simulink model "bhzzz"  (R2016b)
settings: Solver=ode15s  StartTime=0.0  StopTime=60  FixedStep=0.001  RelTol=1e-5  EnableMultiTasking=on
undefined symbols (not defined in the file): b1_damp, b2_damp, b3_damp, b4_damp, g, Hz, L1x, L1y, L1z, L2x, L2y, L2z, L3x, L3y, L3z, mass1, mass2, mass3, mass4, Rturn, theta1_0, theta1_dot_0, theta2_0, theta2_dot_0, theta3_0, theta3_dot_0, theta4_0, theta4_dot_0, X, Y, Z
libraries: sm_lib x50, nesl_utility x34, simulink_extras x2, discretizing x1, simulink x1
(part 2 of 4)

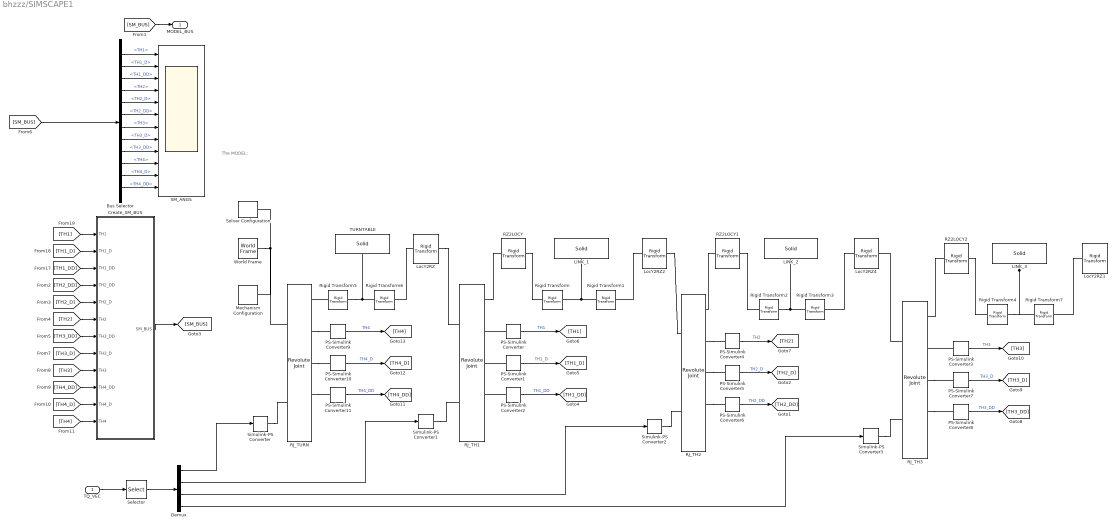
== system bhzzz/SIMSCAPE1 ==
  note: The MODEL:
  TQ_VEC : Inport
  Bus Selector : BusSelector  OutputSignals=TH1,TH1_D,TH1_DD,TH2,TH2_D,TH2_DD,TH3,TH3_D,TH3_DD,TH4,TH4_D,TH4_DD
  Create_SM_BUS : Subsystem
  Demux : Demux
  LINK_1 : sm_lib/Body Elements/Solid  InertiaType=CalculateFromGeometry  Mass=1  MassUnits=kg  CenterOfMass=[0 0 0]  CenterOfMassUnits=m  MomentsOfInertia=[1 1 1]  MomentsOfInertiaUnits=kg*m^2  ProductsOfInertia=[0 0 0]  ProductsOfInertiaUnits=kg*m^2  DensityBased=on  Density=density  DensityUnits=kg/(m^3)  DoExposeReferenceFrame=on  SerializedFrames=<Frames/>  GraphicType=FromGeometry  MarkerShape=Sphere  MarkerSize=10  GraphicVisPropType=SimpleVisualProperties  GraphicDiffuseColor=[0.2 0.2 1.0]  GraphicSpecularColor=[0.5 0.5 0.5 1.0]  GraphicAmbientColor=[0.15 0.15 0.15 1.0]  GraphicEmissiveColor=[0.0 0.0 0.0 1.0]  GraphicShininess=75  GraphicOpacity=1.0  GeometryShape=Brick  RectangleSize=[1 1]  RectangleSizeUnits=m  BrickDimensions=[L1x, L1y, L1z ]  BrickDimensionUnits=m  CylinderRadius=1  CylinderRadiusUnits=m  CylinderLength=1  CylinderLengthUnits=m  SphereRadius=1  SphereRadiusUnits=m  EllipsoidRadii=[1 1 1]  EllipsoidRadiiUnits=m  ExtrusionCrossSection=[1 1; -1 1; -1 -1; 1 -1]  ExtrusionCrossSectionUnits=m  ExtrusionLength=1  ExtrusionLengthUnits=m  PolygonNumSides=3  PolygonOuterRadius=1  PolygonOuterRadiusUnits=m  ExtGeomFileType=STEP  ExtGeomFileUnits=m  RevolutionCrossSection=[1 1; 1 -1; 2 -1; 2 1]  RevolutionCrossSectionUnits=m  RevolutionExtent=Full  RevolutionAngle=180  RevolutionAngleUnits=deg
  LINK_2 : sm_lib/Body Elements/Solid  InertiaType=CalculateFromGeometry  Mass=1  MassUnits=kg  CenterOfMass=[0 0 0]  CenterOfMassUnits=m  MomentsOfInertia=[1 1 1]  MomentsOfInertiaUnits=kg*m^2  ProductsOfInertia=[0 0 0]  ProductsOfInertiaUnits=kg*m^2  DensityBased=on  Density=density  DensityUnits=kg/(m^3)  DoExposeReferenceFrame=on  SerializedFrames=<Frames/>  GraphicType=FromGeometry  MarkerShape=Sphere  MarkerSize=10  GraphicVisPropType=SimpleVisualProperties  GraphicDiffuseColor=[0.8 0.8 1.0]  GraphicSpecularColor=[0.5 0.5 0.5 1.0]  GraphicAmbientColor=[0.15 0.15 0.15 1.0]  GraphicEmissiveColor=[0.0 0.0 0.0 1.0]  GraphicShininess=75  GraphicOpacity=1.0  GeometryShape=Brick  RectangleSize=[1 1]  RectangleSizeUnits=m  BrickDimensions=[L2x, L2y, L2z ]  BrickDimensionUnits=m  CylinderRadius=1  CylinderRadiusUnits=m  CylinderLength=1  CylinderLengthUnits=m  SphereRadius=1  SphereRadiusUnits=m  EllipsoidRadii=[1 1 1]  EllipsoidRadiiUnits=m  ExtrusionCrossSection=[1 1; -1 1; -1 -1; 1 -1]  ExtrusionCrossSectionUnits=m  ExtrusionLength=1  ExtrusionLengthUnits=m  PolygonNumSides=3  PolygonOuterRadius=1  PolygonOuterRadiusUnits=m  ExtGeomFileType=STEP  ExtGeomFileUnits=m  RevolutionCrossSection=[1 1; 1 -1; 2 -1; 2 1]  RevolutionCrossSectionUnits=m  RevolutionExtent=Full  RevolutionAngle=180  RevolutionAngleUnits=deg
  LINK_3 : sm_lib/Body Elements/Solid  InertiaType=CalculateFromGeometry  Mass=1  MassUnits=kg  CenterOfMass=[0 0 0]  CenterOfMassUnits=m  MomentsOfInertia=[1 1 1]  MomentsOfInertiaUnits=kg*m^2  ProductsOfInertia=[0 0 0]  ProductsOfInertiaUnits=kg*m^2  DensityBased=on  Density=density  DensityUnits=kg/(m^3)  DoExposeReferenceFrame=on  SerializedFrames=<Frames/>  GraphicType=FromGeometry  MarkerShape=Sphere  MarkerSize=10  GraphicVisPropType=SimpleVisualProperties  GraphicDiffuseColor=[1.0 0.8 0.4]  GraphicSpecularColor=[0.5 0.5 0.5 1.0]  GraphicAmbientColor=[0.15 0.15 0.15 1.0]  GraphicEmissiveColor=[0.0 0.0 0.0 1.0]  GraphicShininess=75  GraphicOpacity=1.0  GeometryShape=Brick  RectangleSize=[1 1]  RectangleSizeUnits=m  BrickDimensions=[L3x, L3y, L3z ]  BrickDimensionUnits=m  CylinderRadius=1  CylinderRadiusUnits=m  CylinderLength=1  CylinderLengthUnits=m  SphereRadius=1  SphereRadiusUnits=m  EllipsoidRadii=[1 1 1]  EllipsoidRadiiUnits=m  ExtrusionCrossSection=[1 1; -1 1; -1 -1; 1 -1]  ExtrusionCrossSectionUnits=m  ExtrusionLength=1  ExtrusionLengthUnits=m  PolygonNumSides=3  PolygonOuterRadius=1  PolygonOuterRadiusUnits=m  ExtGeomFileType=STEP  ExtGeomFileUnits=m  RevolutionCrossSection=[1 1; 1 -1; 2 -1; 2 1]  RevolutionCrossSectionUnits=m  RevolutionExtent=Full  RevolutionAngle=180  RevolutionAngleUnits=deg
  LocY2RZ{,1..2,4} (4 alike) : sm_lib/Frames and Transforms/Rigid Transform  TranslationMethod=None  TranslationStandardOffset=Hz/2  TranslationLengthUnit=m  TranslationStandardAxis=+Z  TranslationCartesianOffset=[0 0 0]  TranslationROffset=0  TranslationROffsetUnits=m  TranslationZOffset=0  TranslationZOffsetUnits=m  TranslationThetaOffset=0  TranslationThetaOffsetUnits=deg  RotationMethod=AlignedAxes  RotationAngleUnits=deg  RotationStandardAxis=+Z  RotationAngle=0.0  RotationArbitraryAxis=[0 0 1]  FollAlignAxisA=+X  BaseAlignAxisA=+Y  FollAlignAxisB=+Y  BaseAlignAxisB=+Z  RotationSequenceAxes=FollowerAxes  RotationSequence=XYX  RotationSequenceAngles=[0 0 0]  RotationSequenceAnglesUnits=deg  RotationMatrix=[1 0 0; 0 1 0; 0 0 1]
  Mechanism Configuration : sm_lib/Utilities/Mechanism Configuration  UniformGravity=Constant  GravityVector=[0 0 -9.80665 ]  GravityUnits=m/s^2  LinearizationDelta=1e-4
  PS-Simulink Converter{,3..4,9} (4 alike) : nesl_utility/PS-Simulink Converter  PhysicalDomain=network_engine_domain  SubClassName=ps_output  LeftPortType=input  RightPortType=output  PseudoPeriodic=off  Frequencies=[]  Unit=rad  AffineConversion=off
  PS-Simulink Converter{1,5,7,10} (4 alike) : nesl_utility/PS-Simulink Converter  PhysicalDomain=network_engine_domain  SubClassName=ps_output  LeftPortType=input  RightPortType=output  PseudoPeriodic=off  Frequencies=[]  Unit=rad/s  AffineConversion=off
  PS-Simulink Converter{2,6,8,11} (4 alike) : nesl_utility/PS-Simulink Converter  PhysicalDomain=network_engine_domain  SubClassName=ps_output  LeftPortType=input  RightPortType=output  PseudoPeriodic=off  Frequencies=[]  Unit=rad/s^2  AffineConversion=off
  RJ_TH1 : sm_lib/Joints/Revolute Joint  SenseConstraintForce=on  SenseConstraintForceX=off  SenseConstraintForceY=off  SenseConstraintForceZ=off  SenseConstraintTorque=off  SenseConstraintTorqueX=off  SenseConstraintTorqueY=off  SenseConstraintTorqueZ=off  SenseTotalForce=off  SenseTotalForceX=off  SenseTotalForceY=off  SenseTotalForceZ=off  SenseTotalTorque=off  SenseTotalTorqueX=off  SenseTotalTorqueY=off  SenseTotalTorqueZ=off  CompositeWrenchDir=BaseOnFollower  CompositeWrenchFrame=BaseFrame  EquilibriumPosition=0  EquilibriumPositionUnits=deg  SpringStiffness=0  SpringStiffnessUnits=N*m/deg  DampingCoefficient=b1_damp  DampingCoefficientUnits=N*m/(rad/s)  TorqueActuationMode=InputTorque  MotionActuationMode=ComputedMotion  SensePosition=on  SenseVelocity=on  SenseAcceleration=on  SenseTorqueForce=off  PositionTargetSpecify=on  PositionTargetPriority=Low  PositionTargetValue=theta1_0  PositionTargetValueUnits=rad  VelocityTargetSpecify=on  VelocityTargetPriority=High  VelocityTargetValue=theta1_dot_0  VelocityTargetValueUnits=rad/s
      settings: AttributesFormatString=|
      | %<DampingCoefficient>
      | %<PositionTargetValue>
      | %<VelocityTargetValue>
  RJ_TH2 : sm_lib/Joints/Revolute Joint  SenseConstraintForce=on  SenseConstraintForceX=off  SenseConstraintForceY=off  SenseConstraintForceZ=off  SenseConstraintTorque=off  SenseConstraintTorqueX=off  SenseConstraintTorqueY=off  SenseConstraintTorqueZ=off  SenseTotalForce=off  SenseTotalForceX=off  SenseTotalForceY=off  SenseTotalForceZ=off  SenseTotalTorque=off  SenseTotalTorqueX=off  SenseTotalTorqueY=off  SenseTotalTorqueZ=off  CompositeWrenchDir=BaseOnFollower  CompositeWrenchFrame=BaseFrame  EquilibriumPosition=0  EquilibriumPositionUnits=deg  SpringStiffness=0  SpringStiffnessUnits=N*m/deg  DampingCoefficient=b2_damp  DampingCoefficientUnits=N*m/(rad/s)  TorqueActuationMode=InputTorque  MotionActuationMode=ComputedMotion  SensePosition=on  SenseVelocity=on  SenseAcceleration=on  SenseTorqueForce=off  PositionTargetSpecify=on  PositionTargetPriority=Low  PositionTargetValue=theta2_0  PositionTargetValueUnits=rad  VelocityTargetSpecify=on  VelocityTargetPriority=High  VelocityTargetValue=theta2_dot_0  VelocityTargetValueUnits=rad/s
      settings: AttributesFormatString=|
      | %<DampingCoefficient>
      | %<PositionTargetValue>
      | %<VelocityTargetValue>
  RJ_TH3 : sm_lib/Joints/Revolute Joint  SenseConstraintForce=on  SenseConstraintForceX=off  SenseConstraintForceY=off  SenseConstraintForceZ=off  SenseConstraintTorque=off  SenseConstraintTorqueX=off  SenseConstraintTorqueY=off  SenseConstraintTorqueZ=off  SenseTotalForce=off  SenseTotalForceX=off  SenseTotalForceY=off  SenseTotalForceZ=off  SenseTotalTorque=off  SenseTotalTorqueX=off  SenseTotalTorqueY=off  SenseTotalTorqueZ=off  CompositeWrenchDir=BaseOnFollower  CompositeWrenchFrame=BaseFrame  EquilibriumPosition=0  EquilibriumPositionUnits=deg  SpringStiffness=0  SpringStiffnessUnits=N*m/deg  DampingCoefficient=b3_damp  DampingCoefficientUnits=N*m/(rad/s)  TorqueActuationMode=InputTorque  MotionActuationMode=ComputedMotion  SensePosition=on  SenseVelocity=on  SenseAcceleration=on  SenseTorqueForce=off  PositionTargetSpecify=on  PositionTargetPriority=Low  PositionTargetValue=theta3_0  PositionTargetValueUnits=rad  VelocityTargetSpecify=on  VelocityTargetPriority=High  VelocityTargetValue=theta3_dot_0  VelocityTargetValueUnits=rad/s
      settings: AttributesFormatString=|
      | %<DampingCoefficient>
      | %<PositionTargetValue>
      | %<VelocityTargetValue>
  RJ_TURN : sm_lib/Joints/Revolute Joint  SenseConstraintForce=on  SenseConstraintForceX=off  SenseConstraintForceY=off  SenseConstraintForceZ=off  SenseConstraintTorque=off  SenseConstraintTorqueX=off  SenseConstraintTorqueY=off  SenseConstraintTorqueZ=off  SenseTotalForce=off  SenseTotalForceX=off  SenseTotalForceY=off  SenseTotalForceZ=off  SenseTotalTorque=off  SenseTotalTorqueX=off  SenseTotalTorqueY=off  SenseTotalTorqueZ=off  CompositeWrenchDir=BaseOnFollower  CompositeWrenchFrame=BaseFrame  EquilibriumPosition=0  EquilibriumPositionUnits=deg  SpringStiffness=0  SpringStiffnessUnits=N*m/deg  DampingCoefficient=b4_damp  DampingCoefficientUnits=N*m/(rad/s)  TorqueActuationMode=InputTorque  MotionActuationMode=ComputedMotion  SensePosition=on  SenseVelocity=on  SenseAcceleration=on  SenseTorqueForce=off  PositionTargetSpecify=on  PositionTargetPriority=Low  PositionTargetValue=theta4_0  PositionTargetValueUnits=rad  VelocityTargetSpecify=on  VelocityTargetPriority=High  VelocityTargetValue=theta4_dot_0  VelocityTargetValueUnits=rad/s
      settings: AttributesFormatString=|
      | %<DampingCoefficient>
      | %<PositionTargetValue>
      | %<VelocityTargetValue>
  RZ2LOCY : sm_lib/Frames and Transforms/Rigid Transform  TranslationMethod=None  TranslationStandardOffset=Hz/2  TranslationLengthUnit=m  TranslationStandardAxis=+Z  TranslationCartesianOffset=[0 0 0]  TranslationROffset=0  TranslationROffsetUnits=m  TranslationZOffset=0  TranslationZOffsetUnits=m  TranslationThetaOffset=0  TranslationThetaOffsetUnits=deg  RotationMethod=AlignedAxes  RotationAngleUnits=deg  RotationStandardAxis=+Z  RotationAngle=0.0  RotationArbitraryAxis=[0 0 1]  FollAlignAxisA=+Y  BaseAlignAxisA=+X  FollAlignAxisB=+X  BaseAlignAxisB=+Z  RotationSequenceAxes=FollowerAxes  RotationSequence=XYX  RotationSequenceAngles=[0 0 0]  RotationSequenceAnglesUnits=deg  RotationMatrix=[1 0 0; 0 1 0; 0 0 1]
  RZ2LOCY1 : sm_lib/Frames and Transforms/Rigid Transform  TranslationMethod=None  TranslationStandardOffset=Hz/2  TranslationLengthUnit=m  TranslationStandardAxis=+Z  TranslationCartesianOffset=[0 0 0]  TranslationROffset=0  TranslationROffsetUnits=m  TranslationZOffset=0  TranslationZOffsetUnits=m  TranslationThetaOffset=0  TranslationThetaOffsetUnits=deg  RotationMethod=AlignedAxes  RotationAngleUnits=deg  RotationStandardAxis=+Z  RotationAngle=0.0  RotationArbitraryAxis=[0 0 1]  FollAlignAxisA=+Y  BaseAlignAxisA=+X  FollAlignAxisB=+X  BaseAlignAxisB=+Z  RotationSequenceAxes=FollowerAxes  RotationSequence=XYX  RotationSequenceAngles=[0 0 0]  RotationSequenceAnglesUnits=deg  RotationMatrix=[1 0 0; 0 1 0; 0 0 1]
  RZ2LOCY2 : sm_lib/Frames and Transforms/Rigid Transform  TranslationMethod=None  TranslationStandardOffset=Hz/2  TranslationLengthUnit=m  TranslationStandardAxis=+Z  TranslationCartesianOffset=[0 0 0]  TranslationROffset=0  TranslationROffsetUnits=m  TranslationZOffset=0  TranslationZOffsetUnits=m  TranslationThetaOffset=0  TranslationThetaOffsetUnits=deg  RotationMethod=AlignedAxes  RotationAngleUnits=deg  RotationStandardAxis=+Z  RotationAngle=0.0  RotationArbitraryAxis=[0 0 1]  FollAlignAxisA=+Y  BaseAlignAxisA=+X  FollAlignAxisB=+X  BaseAlignAxisB=+Z  RotationSequenceAxes=FollowerAxes  RotationSequence=XYX  RotationSequenceAngles=[0 0 0]  RotationSequenceAnglesUnits=deg  RotationMatrix=[1 0 0; 0 1 0; 0 0 1]
  Rigid Transform : sm_lib/Frames and Transforms/Rigid Transform  TranslationMethod=StandardAxis  TranslationStandardOffset=L1y/2  TranslationLengthUnit=m  TranslationStandardAxis=+Y  TranslationCartesianOffset=[0 0 0]  TranslationROffset=0  TranslationROffsetUnits=m  TranslationZOffset=0  TranslationZOffsetUnits=m  TranslationThetaOffset=0  TranslationThetaOffsetUnits=deg  RotationMethod=None  RotationAngleUnits=deg  RotationStandardAxis=+Z  RotationAngle=0.0  RotationArbitraryAxis=[0 0 1]  FollAlignAxisA=+X  BaseAlignAxisA=+Y  FollAlignAxisB=+Y  BaseAlignAxisB=+Z  RotationSequenceAxes=FollowerAxes  RotationSequence=XYX  RotationSequenceAngles=[0 0 0]  RotationSequenceAnglesUnits=deg  RotationMatrix=[1 0 0; 0 1 0; 0 0 1]
  Rigid Transform1 : sm_lib/Frames and Transforms/Rigid Transform  TranslationMethod=StandardAxis  TranslationStandardOffset=L1y/2  TranslationLengthUnit=m  TranslationStandardAxis=+Y  TranslationCartesianOffset=[0 0 0]  TranslationROffset=0  TranslationROffsetUnits=m  TranslationZOffset=0  TranslationZOffsetUnits=m  TranslationThetaOffset=0  TranslationThetaOffsetUnits=deg  RotationMethod=None  RotationAngleUnits=deg  RotationStandardAxis=+Z  RotationAngle=0.0  RotationArbitraryAxis=[0 0 1]  FollAlignAxisA=+X  BaseAlignAxisA=+Y  FollAlignAxisB=+Y  BaseAlignAxisB=+Z  RotationSequenceAxes=FollowerAxes  RotationSequence=XYX  RotationSequenceAngles=[0 0 0]  RotationSequenceAnglesUnits=deg  RotationMatrix=[1 0 0; 0 1 0; 0 0 1]
  Rigid Transform2 : sm_lib/Frames and Transforms/Rigid Transform  TranslationMethod=StandardAxis  TranslationStandardOffset=L2y/2  TranslationLengthUnit=m  TranslationStandardAxis=+Y  TranslationCartesianOffset=[0 0 0]  TranslationROffset=0  TranslationROffsetUnits=m  TranslationZOffset=0  TranslationZOffsetUnits=m  TranslationThetaOffset=0  TranslationThetaOffsetUnits=deg  RotationMethod=None  RotationAngleUnits=deg  RotationStandardAxis=+Z  RotationAngle=0.0  RotationArbitraryAxis=[0 0 1]  FollAlignAxisA=+X  BaseAlignAxisA=+Y  FollAlignAxisB=+Y  BaseAlignAxisB=+Z  RotationSequenceAxes=FollowerAxes  RotationSequence=XYX  RotationSequenceAngles=[0 0 0]  RotationSequenceAnglesUnits=deg  RotationMatrix=[1 0 0; 0 1 0; 0 0 1]
  Rigid Transform3 : sm_lib/Frames and Transforms/Rigid Transform  TranslationMethod=StandardAxis  TranslationStandardOffset=L2y/2  TranslationLengthUnit=m  TranslationStandardAxis=+Y  TranslationCartesianOffset=[0 0 0]  TranslationROffset=0  TranslationROffsetUnits=m  TranslationZOffset=0  TranslationZOffsetUnits=m  TranslationThetaOffset=0  TranslationThetaOffsetUnits=deg  RotationMethod=None  RotationAngleUnits=deg  RotationStandardAxis=+Z  RotationAngle=0.0  RotationArbitraryAxis=[0 0 1]  FollAlignAxisA=+X  BaseAlignAxisA=+Y  FollAlignAxisB=+Y  BaseAlignAxisB=+Z  RotationSequenceAxes=FollowerAxes  RotationSequence=XYX  RotationSequenceAngles=[0 0 0]  RotationSequenceAnglesUnits=deg  RotationMatrix=[1 0 0; 0 1 0; 0 0 1]
  Rigid Transform4 : sm_lib/Frames and Transforms/Rigid Transform  TranslationMethod=StandardAxis  TranslationStandardOffset=L3y/2  TranslationLengthUnit=m  TranslationStandardAxis=+Y  TranslationCartesianOffset=[0 0 0]  TranslationROffset=0  TranslationROffsetUnits=m  TranslationZOffset=0  TranslationZOffsetUnits=m  TranslationThetaOffset=0  TranslationThetaOffsetUnits=deg  RotationMethod=None  RotationAngleUnits=deg  RotationStandardAxis=+Z  RotationAngle=0.0  RotationArbitraryAxis=[0 0 1]  FollAlignAxisA=+X  BaseAlignAxisA=+Y  FollAlignAxisB=+Y  BaseAlignAxisB=+Z  RotationSequenceAxes=FollowerAxes  RotationSequence=XYX  RotationSequenceAngles=[0 0 0]  RotationSequenceAnglesUnits=deg  RotationMatrix=[1 0 0; 0 1 0; 0 0 1]
  Rigid Transform5 : sm_lib/Frames and Transforms/Rigid Transform  TranslationMethod=StandardAxis  TranslationStandardOffset=Hz/2  TranslationLengthUnit=m  TranslationStandardAxis=-Z  TranslationCartesianOffset=[0 0 0]  TranslationROffset=0  TranslationROffsetUnits=m  TranslationZOffset=0  TranslationZOffsetUnits=m  TranslationThetaOffset=0  TranslationThetaOffsetUnits=deg  RotationMethod=None  RotationAngleUnits=deg  RotationStandardAxis=+Z  RotationAngle=0.0  RotationArbitraryAxis=[0 0 1]  FollAlignAxisA=+X  BaseAlignAxisA=+Y  FollAlignAxisB=+Y  BaseAlignAxisB=+Z  RotationSequenceAxes=FollowerAxes  RotationSequence=XYX  RotationSequenceAngles=[0 0 0]  RotationSequenceAnglesUnits=deg  RotationMatrix=[1 0 0; 0 1 0; 0 0 1]
  Rigid Transform6 : sm_lib/Frames and Transforms/Rigid Transform  TranslationMethod=StandardAxis  TranslationStandardOffset=Hz/2  TranslationLengthUnit=m  TranslationStandardAxis=+Z  TranslationCartesianOffset=[0 0 0]  TranslationROffset=0  TranslationROffsetUnits=m  TranslationZOffset=0  TranslationZOffsetUnits=m  TranslationThetaOffset=0  TranslationThetaOffsetUnits=deg  RotationMethod=None  RotationAngleUnits=deg  RotationStandardAxis=+Z  RotationAngle=0.0  RotationArbitraryAxis=[0 0 1]  FollAlignAxisA=+X  BaseAlignAxisA=+Y  FollAlignAxisB=+Y  BaseAlignAxisB=+Z  RotationSequenceAxes=FollowerAxes  RotationSequence=XYX  RotationSequenceAngles=[0 0 0]  RotationSequenceAnglesUnits=deg  RotationMatrix=[1 0 0; 0 1 0; 0 0 1]
  Rigid Transform7 : sm_lib/Frames and Transforms/Rigid Transform  TranslationMethod=StandardAxis  TranslationStandardOffset=L3y/2  TranslationLengthUnit=m  TranslationStandardAxis=+Y  TranslationCartesianOffset=[0 0 0]  TranslationROffset=0  TranslationROffsetUnits=m  TranslationZOffset=0  TranslationZOffsetUnits=m  TranslationThetaOffset=0  TranslationThetaOffsetUnits=deg  RotationMethod=None  RotationAngleUnits=deg  RotationStandardAxis=+Z  RotationAngle=0.0  RotationArbitraryAxis=[0 0 1]  FollAlignAxisA=+X  BaseAlignAxisA=+Y  FollAlignAxisB=+Y  BaseAlignAxisB=+Z  RotationSequenceAxes=FollowerAxes  RotationSequence=XYX  RotationSequenceAngles=[0 0 0]  RotationSequenceAnglesUnits=deg  RotationMatrix=[1 0 0; 0 1 0; 0 0 1]
  SM_ANGS : Scope  NumInputPorts=12
  Selector : Selector  InputPortWidth=4  IndexOptions=Index vector (dialog)  Indices=[4 1 2 3]  OutputSizes=1
  Simulink-PS Converter{,1..3} (4 alike) : nesl_utility/Simulink-PS Converter  PhysicalDomain=network_engine_domain  SubClassName=ps_input  LeftPortType=input  RightPortType=output  PseudoPeriodic=off  Frequencies=[]  NoiseDistribution=none  NoiseParameters=[]  Unit=N*m  AffineConversion=off  InputFiltering=off  SimscapeFilterOrder=1  InputFilterTimeConstant=0.001  UdotUserProvided=1
  Solver Configuration : nesl_utility/Solver Configuration  PhysicalDomain=network_engine_domain  SubClassName=solver  LeftPortType=input  RightPortType=generic  Accelerate=off  Tones=[]  Harmonics=[]  SimulateNoise=off  Profile=off  UseLocalSampling=off  EnableSwitchedLinearOptims=on  FrequencyDomain=off  UseCCode=off  RelTol=0.001  AbsTol=1e-06  MinStep=1e-09  ToWorkspace=off  RevertToSquareIcSolve=off  NumHomotopyIterations=100  PhasorMode=off  PhasorModeNumHarmonics=1  OverrideAbsTol=off  DoDC=off  ResidualTolerance=1e-09  UseLocalSolver=off  LocalSolverChoice=NE_TRAPEZOIDAL_ADVANCER  LocalSolverSampleTime=0.01  DoFixedCost=off  MaxNonlinIter=3  MaxModeIter=2  LinearAlgebra=Sparse  DelaysMemoryBudget=1024  AutomaticFiltering=off  FilteringTimeConstant=0.001
  TURNTABLE : sm_lib/Body Elements/Solid  InertiaType=CalculateFromGeometry  Mass=1  MassUnits=kg  CenterOfMass=[0 0 0]  CenterOfMassUnits=m  MomentsOfInertia=[1 1 1]  MomentsOfInertiaUnits=kg*m^2  ProductsOfInertia=[0 0 0]  ProductsOfInertiaUnits=kg*m^2  DensityBased=on  Density=1000  DensityUnits=kg/(m^3)  DoExposeReferenceFrame=on  SerializedFrames=<Frames/>  GraphicType=FromGeometry  MarkerShape=Sphere  MarkerSize=10  GraphicVisPropType=SimpleVisualProperties  GraphicDiffuseColor=[1.0 1.0 0.2]  GraphicSpecularColor=[0.5 0.5 0.5 1.0]  GraphicAmbientColor=[0.15 0.15 0.15 1.0]  GraphicEmissiveColor=[0.0 0.0 0.0 1.0]  GraphicShininess=75  GraphicOpacity=1.0  GeometryShape=Cylinder  RectangleSize=[1 1]  RectangleSizeUnits=m  BrickDimensions=[1 1 1]  BrickDimensionUnits=m  CylinderRadius=Rturn  CylinderRadiusUnits=m  CylinderLength=Hz  CylinderLengthUnits=m  SphereRadius=1  SphereRadiusUnits=m  EllipsoidRadii=[1 1 1]  EllipsoidRadiiUnits=m  ExtrusionCrossSection=[1 1; -1 1; -1 -1; 1 -1]  ExtrusionCrossSectionUnits=m  ExtrusionLength=1  ExtrusionLengthUnits=m  PolygonNumSides=3  PolygonOuterRadius=1  PolygonOuterRadiusUnits=m  ExtGeomFileType=STEP  ExtGeomFileUnits=m  RevolutionCrossSection=[1 1; 1 -1; 2 -1; 2 1]  RevolutionCrossSectionUnits=m  RevolutionExtent=Full  RevolutionAngle=180  RevolutionAngleUnits=deg
  World Frame : sm_lib/Frames and Transforms/World Frame
  MODEL_BUS : Outport
  wires:
  [SM_BUS] -> MODEL_BUS/1
  [TH2_D] -> Create_SM_BUS/5(TH2_D)
  [TH1_D] -> Create_SM_BUS/2(TH1_D)
  [TH2_DD] -> Create_SM_BUS/4(TH2_DD)
  [TH2] -> Create_SM_BUS/6(TH2)
  [TH1_DD] -> Create_SM_BUS/3(TH1_DD)
  [TH1] -> Create_SM_BUS/1(TH1)
  Create_SM_BUS/1(SM_BUS) -> [SM_BUS]
  Bus Selector/2 -> SM_ANGS/2  "<TH1_D>"
  Bus Selector/3 -> SM_ANGS/3  "<TH1_DD>"
  Bus Selector/1 -> SM_ANGS/1  "<TH1>"
  Bus Selector/4 -> SM_ANGS/4  "<TH2>"
  Bus Selector/5 -> SM_ANGS/5  "<TH2_D>"
  Bus Selector/6 -> SM_ANGS/6  "<TH2_DD>"
  Bus Selector/7 -> SM_ANGS/7  "<TH3>"
  Bus Selector/8 -> SM_ANGS/8  "<TH3_D>"
  Bus Selector/9 -> SM_ANGS/9  "<TH3_DD>"
  [TH3_DD] -> Create_SM_BUS/7(TH3_DD)
  [TH3_D] -> Create_SM_BUS/8(TH3_D)
  [TH3] -> Create_SM_BUS/9(TH3)
  PS-Simulink Converter/1 -> [TH1]  "TH1"
  PS-Simulink Converter2/1 -> [TH1_DD]  "TH1_DD"
  PS-Simulink Converter1/1 -> [TH1_D]  "TH1_D"
  PS-Simulink Converter4/1 -> [TH2]  "TH2"
  PS-Simulink Converter6/1 -> [TH2_DD]  "TH2_DD"
  PS-Simulink Converter5/1 -> [TH2_D]  "TH2_D"
  PS-Simulink Converter3/1 -> [TH3]  "TH3"
  PS-Simulink Converter8/1 -> [TH3_DD]  "TH3_DD"
  PS-Simulink Converter7/1 -> [TH3_D]  "TH3_D"
  PS-Simulink Converter9/1 -> [TH4]  "TH4"
  PS-Simulink Converter11/1 -> [TH4_DD]  "TH4_DD"
  PS-Simulink Converter10/1 -> [TH4_D]  "TH4_D"
  [TH4_DD] -> Create_SM_BUS/10(TH4_DD)
  [TH4_D] -> Create_SM_BUS/11(TH4_D)
  [TH4] -> Create_SM_BUS/12(TH4)
  Bus Selector/12 -> SM_ANGS/12  "<TH4_DD>"
  Bus Selector/11 -> SM_ANGS/11  "<TH4_D>"
  Bus Selector/10 -> SM_ANGS/10  "<TH4>"
  [SM_BUS] -> Bus Selector/1
  TQ_VEC/1 -> Selector/1
  Selector/1 -> Demux/1
  Demux/1 -> Simulink-PS Converter/1
  Demux/2 -> Simulink-PS Converter1/1
  Demux/3 -> Simulink-PS Converter2/1
  Demux/4 -> Simulink-PS Converter3/1
  connections:
  World Frame/RConn1 -- RJ_TURN/LConn1 -- Mechanism Configuration/RConn1 -- Solver Configuration/RConn1
  PS-Simulink Converter1/LConn1 -- RJ_TH1/RConn3
  PS-Simulink Converter2/LConn1 -- RJ_TH1/RConn4
  PS-Simulink Converter/LConn1 -- RJ_TH1/RConn2
  Rigid Transform5/LConn1 -- RJ_TURN/RConn1
  Rigid Transform5/RConn1 -- Rigid Transform6/LConn1 -- TURNTABLE/RConn1
  LocY2RZ/LConn1 -- Rigid Transform6/RConn1
  LocY2RZ/RConn1 -- RJ_TH1/LConn1
  Rigid Transform1/LConn1 -- LINK_1/RConn1 -- Rigid Transform/RConn1
  LocY2RZ2/LConn1 -- Rigid Transform1/RConn1
  LocY2RZ2/RConn1 -- RJ_TH2/LConn1
  RZ2LOCY1/LConn1 -- RJ_TH2/RConn1
  Rigid Transform2/RConn1 -- Rigid Transform3/LConn1 -- LINK_2/RConn1
  LocY2RZ4/LConn1 -- Rigid Transform3/RConn1
  RJ_TH1/RConn1 -- RZ2LOCY/LConn1
  RZ2LOCY/RConn1 -- Rigid Transform/LConn1
  RZ2LOCY1/RConn1 -- Rigid Transform2/LConn1
  RJ_TH3/LConn1 -- LocY2RZ4/RConn1
  LINK_3/RConn1 -- Rigid Transform7/LConn1 -- Rigid Transform4/RConn1
  LocY2RZ1/LConn1 -- Rigid Transform7/RConn1
  RZ2LOCY2/RConn1 -- Rigid Transform4/LConn1
  RZ2LOCY2/LConn1 -- RJ_TH3/RConn1
  RJ_TH2/RConn3 -- PS-Simulink Converter5/LConn1
  RJ_TH2/RConn2 -- PS-Simulink Converter4/LConn1
  RJ_TH2/RConn4 -- PS-Simulink Converter6/LConn1
  PS-Simulink Converter3/LConn1 -- RJ_TH3/RConn2
  RJ_TH3/RConn3 -- PS-Simulink Converter7/LConn1
  RJ_TH3/RConn4 -- PS-Simulink Converter8/LConn1
  RJ_TURN/RConn4 -- PS-Simulink Converter11/LConn1
  RJ_TURN/RConn3 -- PS-Simulink Converter10/LConn1
  RJ_TURN/RConn2 -- PS-Simulink Converter9/LConn1
  Simulink-PS Converter/RConn1 -- RJ_TURN/LConn2
  Simulink-PS Converter2/RConn1 -- RJ_TH2/LConn2
  Simulink-PS Converter3/RConn1 -- RJ_TH3/LConn2
  Simulink-PS Converter1/RConn1 -- RJ_TH1/LConn2

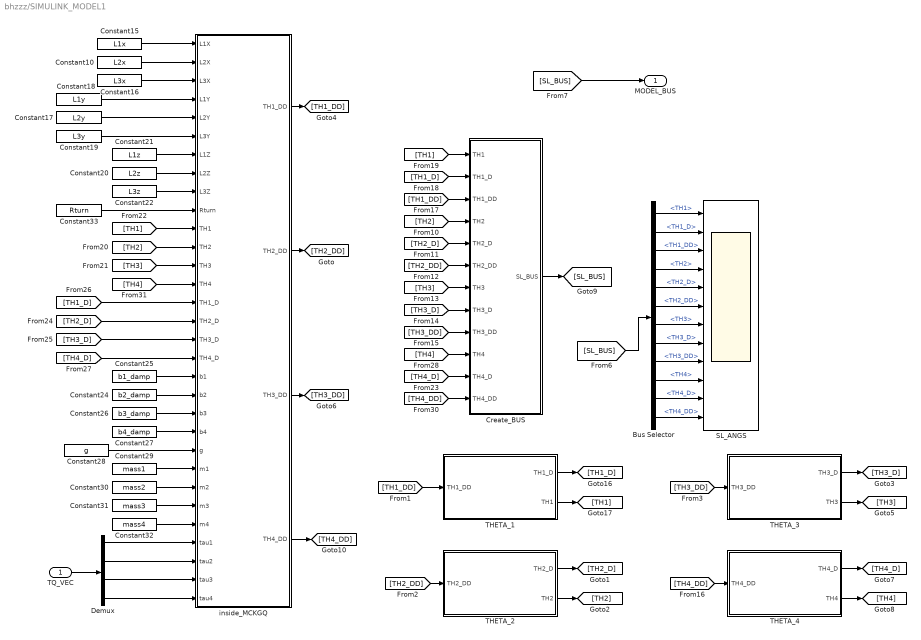
== system bhzzz/SIMULINK_MODEL1 ==
  TQ_VEC : Inport
  Bus Selector : BusSelector  OutputSignals=TH1,TH1_D,TH1_DD,TH2,TH2_D,TH2_DD,TH3,TH3_D,TH3_DD,TH4,TH4_D,TH4_DD
  Constant10 : Constant  Value=L2x
  Constant15 : Constant  Value=L1x
  Constant16 : Constant  Value=L3x
  Constant17 : Constant  Value=L2y
  Constant18 : Constant  Value=L1y
  Constant19 : Constant  Value=L3y
  Constant20 : Constant  Value=L2z
  Constant21 : Constant  Value=L1z
  Constant22 : Constant  Value=L3z
  Constant24 : Constant  Value=b2_damp
  Constant25 : Constant  Value=b1_damp
  Constant26 : Constant  Value=b3_damp
  Constant27 : Constant  Value=b4_damp
  Constant28 : Constant  Value=g
  Constant29 : Constant  Value=mass1
  Constant30 : Constant  Value=mass2
  Constant31 : Constant  Value=mass3
  Constant32 : Constant  Value=mass4
  Constant33 : Constant  Value=Rturn
  Create_BUS : Subsystem
  Demux : Demux
  SL_ANGS : Scope  NumInputPorts=12
  THETA_1 : Subsystem
  THETA_2 : Subsystem
  THETA_3 : Subsystem
  THETA_4 : Subsystem
  inside_MCKGQ : Subsystem
  MODEL_BUS : Outport
  wires:
  [SL_BUS] -> Bus Selector/1
  Create_BUS/1(SL_BUS) -> [SL_BUS]
  Bus Selector/2 -> SL_ANGS/2  "<TH1_D>"
  Bus Selector/3 -> SL_ANGS/3  "<TH1_DD>"
  Bus Selector/1 -> SL_ANGS/1  "<TH1>"
  Bus Selector/4 -> SL_ANGS/4  "<TH2>"
  Bus Selector/5 -> SL_ANGS/5  "<TH2_D>"
  Bus Selector/6 -> SL_ANGS/6  "<TH2_DD>"
  Bus Selector/7 -> SL_ANGS/7  "<TH3>"
  Bus Selector/8 -> SL_ANGS/8  "<TH3_D>"
  Bus Selector/9 -> SL_ANGS/9  "<TH3_DD>"
  [TH2_DD] -> THETA_2/1(TH2_DD)
  THETA_2/2(TH2) -> [TH2]
  THETA_2/1(TH2_D) -> [TH2_D]
  [TH1_DD] -> THETA_1/1(TH1_DD)
  THETA_1/1(TH1_D) -> [TH1_D]
  THETA_1/2(TH1) -> [TH1]
  inside_MCKGQ/2(TH2_DD) -> [TH2_DD]
  [TH3_DD] -> THETA_3/1(TH3_DD)
  THETA_3/2(TH3) -> [TH3]
  THETA_3/1(TH3_D) -> [TH3_D]
  inside_MCKGQ/1(TH1_DD) -> [TH1_DD]
  inside_MCKGQ/3(TH3_DD) -> [TH3_DD]
  [TH3_DD] -> Create_BUS/9(TH3_DD)
  [TH1] -> Create_BUS/1(TH1)
  [TH1_D] -> Create_BUS/2(TH1_D)
  [TH1_DD] -> Create_BUS/3(TH1_DD)
  [TH2] -> Create_BUS/4(TH2)
  [TH2_D] -> Create_BUS/5(TH2_D)
  [TH2_DD] -> Create_BUS/6(TH2_DD)
  [TH3] -> Create_BUS/7(TH3)
  [TH3_D] -> Create_BUS/8(TH3_D)
  [TH4_DD] -> THETA_4/1(TH4_DD)
  THETA_4/2(TH4) -> [TH4]
  THETA_4/1(TH4_D) -> [TH4_D]
  [TH2] -> inside_MCKGQ/12(TH2)
  [TH3] -> inside_MCKGQ/13(TH3)
  [TH1] -> inside_MCKGQ/11(TH1)
  Constant10/1 -> inside_MCKGQ/2(L2X)
  Constant16/1 -> inside_MCKGQ/3(L3X)
  Constant15/1 -> inside_MCKGQ/1(L1X)
  Constant19/1 -> inside_MCKGQ/6(L3Y)
  Constant17/1 -> inside_MCKGQ/5(L2Y)
  Constant18/1 -> inside_MCKGQ/4(L1Y)
  Constant22/1 -> inside_MCKGQ/9(L3Z)
  Constant20/1 -> inside_MCKGQ/8(L2Z)
  Constant21/1 -> inside_MCKGQ/7(L1Z)
  [TH1_D] -> inside_MCKGQ/15(TH1_D)
  [TH2_D] -> inside_MCKGQ/16(TH2_D)
  [TH3_D] -> inside_MCKGQ/17(TH3_D)
  [TH4_D] -> inside_MCKGQ/18(TH4_D)
  Constant25/1 -> inside_MCKGQ/19(b1)
  Constant24/1 -> inside_MCKGQ/20(b2)
  Constant26/1 -> inside_MCKGQ/21(b3)
  Constant27/1 -> inside_MCKGQ/22(b4)
  Constant28/1 -> inside_MCKGQ/23(g)
  Constant29/1 -> inside_MCKGQ/24(m1)
  Constant30/1 -> inside_MCKGQ/25(m2)
  Constant31/1 -> inside_MCKGQ/26(m3)
  Constant32/1 -> inside_MCKGQ/27(m4)
  Constant33/1 -> inside_MCKGQ/10(Rturn)
  [TH4_D] -> Create_BUS/11(TH4_D)
  [TH4_DD] -> Create_BUS/12(TH4_DD)
  [TH4] -> Create_BUS/10(TH4)
  [TH4] -> inside_MCKGQ/14(TH4)
  inside_MCKGQ/4(TH4_DD) -> [TH4_DD]
  Bus Selector/10 -> SL_ANGS/10  "<TH4>"
  Bus Selector/11 -> SL_ANGS/11  "<TH4_D>"
  Bus Selector/12 -> SL_ANGS/12  "<TH4_DD>"
  [SL_BUS] -> MODEL_BUS/1
  Demux/1 -> inside_MCKGQ/28(tau1)
  Demux/2 -> inside_MCKGQ/29(tau2)
  Demux/3 -> inside_MCKGQ/30(tau3)
  Demux/4 -> inside_MCKGQ/31(tau4)
  TQ_VEC/1 -> Demux/1

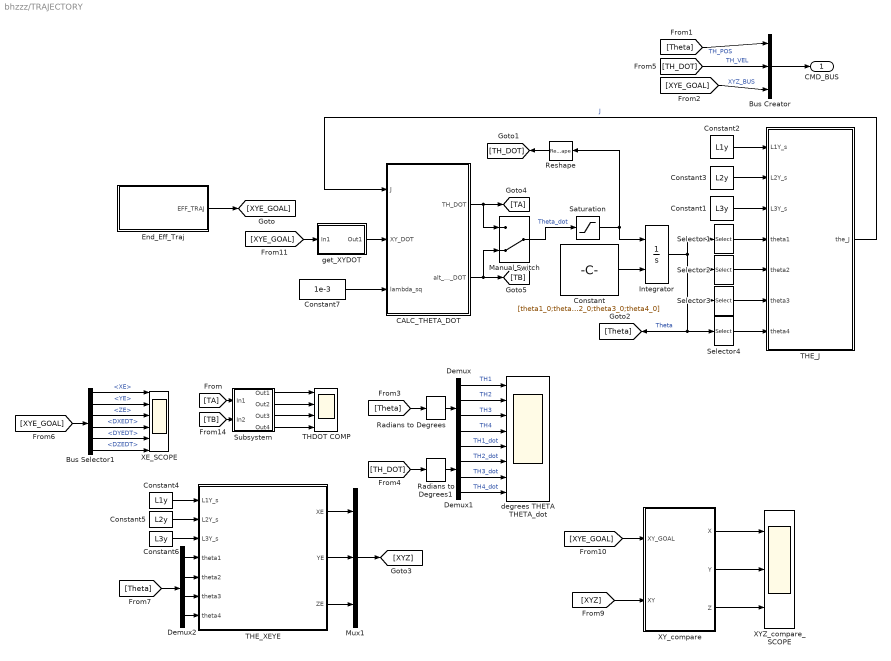
== system bhzzz/TRAJECTORY ==
  Bus Creator : BusCreator  Inputs=3
  Bus Selector1 : BusSelector  OutputSignals=XE,YE,ZE,DXEDT,DYEDT,DZEDT
  CALC_THETA_DOT : MATLAB Function  TreatAsAtomicUnit=on
  Constant : Constant  Value=[theta1_0;theta2_0;theta3_0;theta4_0]  VectorParams1D=off
  Constant1 : Constant  Value=L3y
  Constant2 : Constant  Value=L1y
  Constant3 : Constant  Value=L2y
  Constant4 : Constant  Value=L1y
  Constant5 : Constant  Value=L2y
  Constant6 : Constant  Value=L3y
  Constant7 : Constant  Value=1e-3
  Demux : Demux
  Demux1 : Demux
  Demux2 : Demux
  End_Eff_Traj : Subsystem
  Integrator : Integrator  InitialConditionSource=external
  Manual Switch : ManualSwitch  CurrentSetting=0
  Mux1 : Mux  Inputs=3
  Radians to Degrees : simulink_extras/Transformations/Radians to Degrees
  Radians to Degrees1 : simulink_extras/Transformations/Radians to Degrees
  Reshape : Reshape  OutputDimensionality=Column vector (2-D)
  Saturation : Saturate  UpperLimit=6  LowerLimit=-6
  Selector1 : Selector  InputPortWidth=4  IndexOptions=Index vector (dialog)  Indices=1  OutputSizes=1
  Selector2 : Selector  InputPortWidth=4  IndexOptions=Index vector (dialog)  Indices=2  OutputSizes=1
  Selector3 : Selector  InputPortWidth=4  IndexOptions=Index vector (dialog)  Indices=3  OutputSizes=1
  Selector4 : Selector  InputPortWidth=4  IndexOptions=Index vector (dialog)  Indices=4  OutputSizes=1
  Subsystem : Subsystem
  THDOT COMP : Scope  NumInputPorts=4
  THE_J : MATLAB Function  TreatAsAtomicUnit=on
  THE_XEYE : MATLAB Function  TreatAsAtomicUnit=on
  XE_SCOPE : Scope  NumInputPorts=6
  XYZ_compare_SCOPE : Scope  NumInputPorts=3
  XY_compare : Subsystem
  degrees THETA THETA_dot : Scope  NumInputPorts=8
  get_XYDOT : Subsystem
  CMD_BUS : Outport
  wires:
  Bus Selector1/1 -> XE_SCOPE/1  "<XE>"
  Bus Selector1/2 -> XE_SCOPE/2  "<YE>"
  Bus Selector1/3 -> XE_SCOPE/3  "<ZE>"
  Bus Selector1/4 -> XE_SCOPE/4  "<DXEDT>"
  Bus Selector1/5 -> XE_SCOPE/5  "<DYEDT>"
  Bus Selector1/6 -> XE_SCOPE/6  "<DZEDT>"
  [XYE_GOAL] -> Bus Selector1/1
  Constant/1 -> Integrator/2
  THE_J/1(the_J) -> CALC_THETA_DOT/1(J)  "J"
  get_XYDOT/1(Out1) -> CALC_THETA_DOT/2(XY_DOT)
  Manual Switch/1 -> Saturation/1  "Theta_dot"
  Integrator/1 -> Selector4/1, [Theta], Selector3/1, Selector2/1, Selector1/1  "Theta"
  [XYE_GOAL] -> get_XYDOT/1(In1)
  Saturation/1 -> Integrator/1, Reshape/1
  Selector4/1 -> THE_J/7(theta4)
  Selector3/1 -> THE_J/6(theta3)
  Selector2/1 -> THE_J/5(theta2)
  Selector1/1 -> THE_J/4(theta1)
  Constant2/1 -> THE_J/1(L1Y_s)
  Constant3/1 -> THE_J/2(L2Y_s)
  Constant1/1 -> THE_J/3(L3Y_s)
  CALC_THETA_DOT/1(TH_DOT) -> [TA], Manual Switch/1
  CALC_THETA_DOT/2(alt_TH_DOT) -> [TB], Manual Switch/2
  Constant7/1 -> CALC_THETA_DOT/3(lambda_sq)
  [TB] -> Subsystem/2(In2)
  [TA] -> Subsystem/1(In1)
  Subsystem/1(Out1) -> THDOT COMP/1
  Subsystem/2(Out2) -> THDOT COMP/2
  Subsystem/3(Out3) -> THDOT COMP/3
  Subsystem/4(Out4) -> THDOT COMP/4
  End_Eff_Traj/1(EFF_TRAJ) -> [XYE_GOAL]
  [TH_DOT] -> Bus Creator/2  "TH_VEL"
  [Theta] -> Bus Creator/1  "TH_POS"
  Bus Creator/1 -> CMD_BUS/1
  Reshape/1 -> [TH_DOT]
  [XYE_GOAL] -> Bus Creator/3  "XYZ_BUS"
  Demux/4 -> degrees THETA THETA_dot/4  "TH4"
  Demux/3 -> degrees THETA THETA_dot/3  "TH3"
  Demux/2 -> degrees THETA THETA_dot/2  "TH2"
  Demux/1 -> degrees THETA THETA_dot/1  "TH1"
  Demux1/1 -> degrees THETA THETA_dot/5  "TH1_dot"
  Demux1/2 -> degrees THETA THETA_dot/6  "TH2_dot"
  Demux1/3 -> degrees THETA THETA_dot/7  "TH3_dot"
  Demux1/4 -> degrees THETA THETA_dot/8  "TH4_dot"
  [Theta] -> Radians to Degrees/1
  Radians to Degrees/1 -> Demux/1
  [TH_DOT] -> Radians to Degrees1/1
  Radians to Degrees1/1 -> Demux1/1
  Constant4/1 -> THE_XEYE/1(L1Y_s)
  Constant6/1 -> THE_XEYE/3(L3Y_s)
  Constant5/1 -> THE_XEYE/2(L2Y_s)
  Demux2/1 -> THE_XEYE/4(theta1)
  Demux2/2 -> THE_XEYE/5(theta2)
  Demux2/3 -> THE_XEYE/6(theta3)
  Demux2/4 -> THE_XEYE/7(theta4)
  [Theta] -> Demux2/1
  THE_XEYE/1(XE) -> Mux1/1
  THE_XEYE/3(ZE) -> Mux1/3
  THE_XEYE/2(YE) -> Mux1/2
  Mux1/1 -> [XYZ]
  [XYZ] -> XY_compare/2(XY)
  XY_compare/2(Y) -> XYZ_compare_SCOPE/2
  XY_compare/1(X) -> XYZ_compare_SCOPE/1
  [XYE_GOAL] -> XY_compare/1(XY_GOAL)
  XY_compare/3(Z) -> XYZ_compare_SCOPE/3

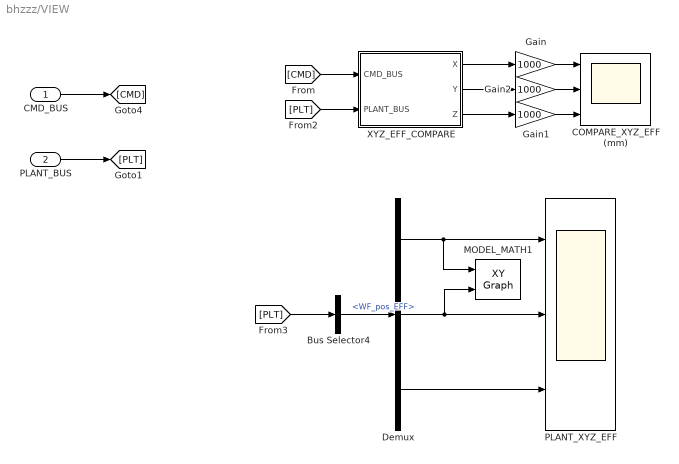
== system bhzzz/VIEW ==
  CMD_BUS : Inport
  PLANT_BUS : Inport  Port=2
  Bus Selector4 : BusSelector  OutputSignals=CALC_POS_BUS.WF_pos_EFF
  COMPARE_XYZ_EFF (mm) : Scope  NumInputPorts=3
  Demux : Demux  Outputs=3
  Gain : Gain  Gain=1000
  Gain1 : Gain  Gain=1000
  Gain2 : Gain  Gain=1000
  MODEL_MATH1 : simulink/Sinks/XY Graph  xmin=0  xmax=1.6  ymin=0  ymax=1.6  st=-1
  PLANT_XYZ_EFF : Scope  NumInputPorts=3
  XYZ_EFF_COMPARE : Subsystem
  wires:
  CMD_BUS/1 -> [CMD]
  PLANT_BUS/1 -> [PLT]
  [CMD] -> XYZ_EFF_COMPARE/1(CMD_BUS)
  [PLT] -> XYZ_EFF_COMPARE/2(PLANT_BUS)
  XYZ_EFF_COMPARE/1(X) -> Gain/1
  XYZ_EFF_COMPARE/2(Y) -> Gain2/1
  XYZ_EFF_COMPARE/3(Z) -> Gain1/1
  Bus Selector4/1 -> Demux/1  "<WF_pos_EFF>"
  Demux/1 -> MODEL_MATH1/1, PLANT_XYZ_EFF/1
  Demux/2 -> MODEL_MATH1/2, PLANT_XYZ_EFF/2
  [PLT] -> Bus Selector4/1
  Demux/3 -> PLANT_XYZ_EFF/3
  Gain/1 -> COMPARE_XYZ_EFF (mm)/1
  Gain1/1 -> COMPARE_XYZ_EFF (mm)/3
  Gain2/1 -> COMPARE_XYZ_EFF (mm)/2

== system bhzzz/Create_PLANT_BUS1/CALC_BUS ==
  MODEL_BUS : Inport
  Bus Creator : BusCreator  Inputs=14
  Bus Selector : BusSelector  OutputSignals=TH1,TH2,TH3,TH4
  Bus Selector1 : BusSelector  OutputSignals=TH1,TH2,TH3
  Constant1 : Constant  Value=L2y
  Constant17 : Constant  Value=L2y
  Constant18 : Constant  Value=L1y
  Constant19 : Constant  Value=L3y
  Constant2 : Constant  Value=L1y
  Constant3 : Constant  Value=L3y
  THE_A_EFF_and_O_and_G : MATLAB Function  TreatAsAtomicUnit=on
  THE_W_EFF_and_O_and_G : MATLAB Function  TreatAsAtomicUnit=on
  CALC_POS : Outport
  wires:
  Bus Selector/1 -> THE_W_EFF_and_O_and_G/4(theta1)  "<TH1>"
  Bus Selector/2 -> THE_W_EFF_and_O_and_G/5(theta2)  "<TH2>"
  Bus Selector/3 -> THE_W_EFF_and_O_and_G/6(theta3)  "<TH3>"
  Bus Selector/4 -> THE_W_EFF_and_O_and_G/7(theta4)  "<TH4>"
  Bus Creator/1 -> CALC_POS/1
  Constant18/1 -> THE_W_EFF_and_O_and_G/1(L1Y_s)
  Constant17/1 -> THE_W_EFF_and_O_and_G/2(L2Y_s)
  Constant19/1 -> THE_W_EFF_and_O_and_G/3(L3Y_s)
  THE_W_EFF_and_O_and_G/4(WF_pos_O3) -> Bus Creator/4  "WF_pos_O3"
  THE_W_EFF_and_O_and_G/6(WF_pos_G2) -> Bus Creator/6  "WF_pos_G2"
  THE_W_EFF_and_O_and_G/3(WF_pos_O2) -> Bus Creator/3  "WF_pos_O2"
  THE_W_EFF_and_O_and_G/7(WF_pos_G3) -> Bus Creator/7  "WF_pos_G3"
  THE_W_EFF_and_O_and_G/1(WF_pos_eff) -> Bus Creator/1  "WF_pos_EFF"
  THE_W_EFF_and_O_and_G/5(WF_pos_G1) -> Bus Creator/5  "WF_pos_G1"
  THE_W_EFF_and_O_and_G/2(WF_pos_O1) -> Bus Creator/2  "WF_pos_O1"
  MODEL_BUS/1 -> Bus Selector1/1, Bus Selector/1
  Bus Selector1/1 -> THE_A_EFF_and_O_and_G/4(theta1)  "<TH1>"
  Bus Selector1/2 -> THE_A_EFF_and_O_and_G/5(theta2)  "<TH2>"
  Bus Selector1/3 -> THE_A_EFF_and_O_and_G/6(theta3)  "<TH3>"
  Constant2/1 -> THE_A_EFF_and_O_and_G/1(L1Y_s)
  Constant1/1 -> THE_A_EFF_and_O_and_G/2(L2Y_s)
  Constant3/1 -> THE_A_EFF_and_O_and_G/3(L3Y_s)
  THE_A_EFF_and_O_and_G/7(AF_pos_G3) -> Bus Creator/14  "AF_pos_G3"
  THE_A_EFF_and_O_and_G/6(AF_pos_G2) -> Bus Creator/13  "AF_pos_G2"
  THE_A_EFF_and_O_and_G/5(AF_pos_G1) -> Bus Creator/12  "AF_pos_G1"
  THE_A_EFF_and_O_and_G/4(AF_pos_O3) -> Bus Creator/11  "AF_pos_O3"
  THE_A_EFF_and_O_and_G/3(AF_pos_O2) -> Bus Creator/10  "AF_pos_O2"
  THE_A_EFF_and_O_and_G/2(AF_pos_O1) -> Bus Creator/9  "AF_pos_O1"
  THE_A_EFF_and_O_and_G/1(AF_pos_eff) -> Bus Creator/8  "AF_pos_EFF"

== system bhzzz/Create_PLANT_BUS1/MEAS ==
  MODEL_BUS : Inport
  Bus Creator : BusCreator  Inputs=3
  Bus Selector : BusSelector  OutputSignals=TH1,TH2,TH3,TH4
  Bus Selector1 : BusSelector  OutputSignals=TH1_D,TH2_D,TH3_D,TH4_D
  Bus Selector2 : BusSelector  OutputSignals=TH1_DD,TH2_DD,TH3_DD,TH4_DD
  Mux : Mux
  Mux1 : Mux
  Mux2 : Mux
  Reshape : Reshape  OutputDimensionality=Column vector (2-D)
  Reshape1 : Reshape  OutputDimensionality=Column vector (2-D)
  Reshape2 : Reshape  OutputDimensionality=Column vector (2-D)
  MEAS : Outport
  wires:
  MODEL_BUS/1 -> Bus Selector/1, Bus Selector2/1, Bus Selector1/1
  Bus Selector/1 -> Mux/1  "<TH1>"
  Bus Selector/2 -> Mux/2  "<TH2>"
  Bus Selector/3 -> Mux/3  "<TH3>"
  Bus Selector/4 -> Mux/4  "<TH4>"
  Bus Selector1/1 -> Mux1/1  "<TH1_D>"
  Bus Selector1/2 -> Mux1/2  "<TH2_D>"
  Bus Selector1/3 -> Mux1/3  "<TH3_D>"
  Bus Selector1/4 -> Mux1/4  "<TH4_D>"
  Bus Selector2/1 -> Mux2/1  "<TH1_DD>"
  Bus Selector2/2 -> Mux2/2  "<TH2_DD>"
  Bus Selector2/3 -> Mux2/3  "<TH3_DD>"
  Bus Selector2/4 -> Mux2/4  "<TH4_DD>"
  Mux/1 -> Reshape/1  "TH_POS"
  Mux1/1 -> Reshape1/1  "TH_VEL"
  Mux2/1 -> Reshape2/1  "TH_ACC"
  Reshape/1 -> Bus Creator/1  "TH_POS"
  Reshape1/1 -> Bus Creator/2  "TH_VEL"
  Reshape2/1 -> Bus Creator/3  "TH_ACC"
  Bus Creator/1 -> MEAS/1

== system bhzzz/Create_PLANT_BUS1/Subsystem ==
  MODEL : Inport
  MEAS : Inport  Port=2
  CALC_POS : Inport  Port=3
  CALC_GRAV_TQ : Inport  Port=4
  Bus Creator : BusCreator  Inputs=4
  PLANT_B : Outport
  wires:
  MODEL/1 -> Bus Creator/1  "MODEL_BUS"
  MEAS/1 -> Bus Creator/2  "MEAS_BUS"
  CALC_POS/1 -> Bus Creator/3  "CALC_POS_BUS"
  Bus Creator/1 -> PLANT_B/1
  CALC_GRAV_TQ/1 -> Bus Creator/4  "CALC_GRAV_TQ_BUS"

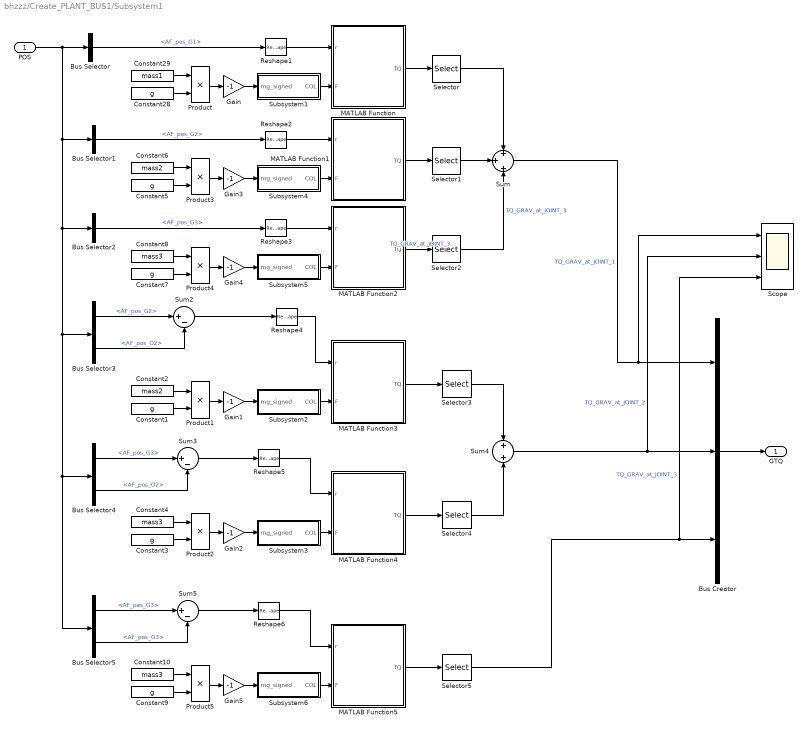
== system bhzzz/Create_PLANT_BUS1/Subsystem1 ==
  POS : Inport
  Bus Creator : BusCreator  Inputs=3
  Bus Selector : BusSelector  OutputSignals=AF_pos_G1
  Bus Selector1 : BusSelector  OutputSignals=AF_pos_G2
  Bus Selector2 : BusSelector  OutputSignals=AF_pos_G3
  Bus Selector3 : BusSelector  OutputSignals=AF_pos_G2,AF_pos_O2
  Bus Selector4 : BusSelector  OutputSignals=AF_pos_G3,AF_pos_O2
  Bus Selector5 : BusSelector  OutputSignals=AF_pos_G3,AF_pos_O3
  Constant{1,3,5,7,9,28} (6 alike) : Constant  Value=g
  Constant10 : Constant  Value=mass3
  Constant2 : Constant  Value=mass2
  Constant29 : Constant  Value=mass1
  Constant4 : Constant  Value=mass3
  Constant6 : Constant  Value=mass2
  Constant8 : Constant  Value=mass3
  Gain{,1..5} (6 alike) : Gain  Gain=-1
  MATLAB Function : MATLAB Function  TreatAsAtomicUnit=on
  MATLAB Function1 : MATLAB Function  TreatAsAtomicUnit=on
  MATLAB Function2 : MATLAB Function  TreatAsAtomicUnit=on
  MATLAB Function3 : MATLAB Function  TreatAsAtomicUnit=on
  MATLAB Function4 : MATLAB Function  TreatAsAtomicUnit=on
  MATLAB Function5 : MATLAB Function  TreatAsAtomicUnit=on
  Product{,1..5} (6 alike) : Product
  Reshape{1..6} (6 alike) : Reshape  OutputDimensionality=Column vector (2-D)
  Scope : Scope  NumInputPorts=3
  Selector{,1..5} (6 alike) : Selector  InputPortWidth=3  IndexOptions=Index vector (dialog)  Indices=1  OutputSizes=1
  Subsystem1 : Subsystem
  Subsystem2 : Subsystem
  Subsystem3 : Subsystem
  Subsystem4 : Subsystem
  Subsystem5 : Subsystem
  Subsystem6 : Subsystem
  Sum : Sum  Inputs=+|+|+
  Sum2 : Sum  Inputs=|+-
  Sum3 : Sum  Inputs=|+-
  Sum4 : Sum  Inputs=+|+
  Sum5 : Sum  Inputs=|+-
  GTQ : Outport
  wires:
  Bus Selector/1 -> Reshape1/1  "<AF_pos_G1>"
  Constant29/1 -> Product/1
  Constant28/1 -> Product/2
  Product/1 -> Gain/1
  Gain/1 -> Subsystem1/1(mg_signed)
  Subsystem1/1(COL) -> MATLAB Function/2(F)
  Reshape1/1 -> MATLAB Function/1(r)
  Bus Selector1/1 -> Reshape2/1  "<AF_pos_G2>"
  Constant6/1 -> Product3/1
  Constant5/1 -> Product3/2
  Product3/1 -> Gain3/1
  Gain3/1 -> Subsystem4/1(mg_signed)
  Subsystem4/1(COL) -> MATLAB Function1/2(F)
  Reshape2/1 -> MATLAB Function1/1(r)
  Bus Selector2/1 -> Reshape3/1  "<AF_pos_G3>"
  Constant8/1 -> Product4/1
  Constant7/1 -> Product4/2
  Product4/1 -> Gain4/1
  Gain4/1 -> Subsystem5/1(mg_signed)
  Subsystem5/1(COL) -> MATLAB Function2/2(F)
  Reshape3/1 -> MATLAB Function2/1(r)
  MATLAB Function/1(TQ) -> Selector/1
  MATLAB Function2/1(TQ) -> Selector2/1  "TQ_GRAV_at_JOINT_3"
  MATLAB Function1/1(TQ) -> Selector1/1
  Bus Creator/1 -> GTQ/1
  Selector/1 -> Sum/1
  Selector1/1 -> Sum/2
  Selector2/1 -> Sum/3  "TQ_GRAV_at_JOINT_3"
  Bus Selector3/1 -> Sum2/1  "<AF_pos_G2>"
  Constant2/1 -> Product1/1
  Constant1/1 -> Product1/2
  Product1/1 -> Gain1/1
  Gain1/1 -> Subsystem2/1(mg_signed)
  Subsystem2/1(COL) -> MATLAB Function3/2(F)
  Reshape4/1 -> MATLAB Function3/1(r)
  Bus Selector4/1 -> Sum3/1  "<AF_pos_G3>"
  Constant4/1 -> Product2/1
  Constant3/1 -> Product2/2
  Product2/1 -> Gain2/1
  Gain2/1 -> Subsystem3/1(mg_signed)
  Subsystem3/1(COL) -> MATLAB Function4/2(F)
  Reshape5/1 -> MATLAB Function4/1(r)
  Sum2/1 -> Reshape4/1
  Bus Selector3/2 -> Sum2/2  "<AF_pos_O2>"
  Bus Selector4/2 -> Sum3/2  "<AF_pos_O2>"
  Sum3/1 -> Reshape5/1
  MATLAB Function3/1(TQ) -> Selector3/1
  MATLAB Function4/1(TQ) -> Selector4/1
  Selector3/1 -> Sum4/1
  Selector4/1 -> Sum4/2
  POS/1 -> Bus Selector5/1, Bus Selector4/1, Bus Selector3/1, Bus Selector2/1, Bus Selector1/1, Bus Selector/1
  Bus Selector5/1 -> Sum5/1  "<AF_pos_G3>"
  Constant10/1 -> Product5/1
  Constant9/1 -> Product5/2
  Product5/1 -> Gain5/1
  Gain5/1 -> Subsystem6/1(mg_signed)
  Subsystem6/1(COL) -> MATLAB Function5/2(F)
  Reshape6/1 -> MATLAB Function5/1(r)
  Bus Selector5/2 -> Sum5/2  "<AF_pos_O3>"
  Sum5/1 -> Reshape6/1
  MATLAB Function5/1(TQ) -> Selector5/1
  Sum4/1 -> Scope/2, Bus Creator/2  "TQ_GRAV_at_JOINT_2"
  Sum/1 -> Scope/1, Bus Creator/1  "TQ_GRAV_at_JOINT_1"
  Selector5/1 -> Scope/3, Bus Creator/3  "TQ_GRAV_at_JOINT_3"

== system bhzzz/Create_PLANT_BUS2/CALC_BUS ==
  MODEL_BUS : Inport
  Bus Creator : BusCreator  Inputs=14
  Bus Selector : BusSelector  OutputSignals=TH1,TH2,TH3,TH4
  Bus Selector1 : BusSelector  OutputSignals=TH1,TH2,TH3
  Constant1 : Constant  Value=L2y
  Constant17 : Constant  Value=L2y
  Constant18 : Constant  Value=L1y
  Constant19 : Constant  Value=L3y
  Constant2 : Constant  Value=L1y
  Constant3 : Constant  Value=L3y
  THE_A_EFF_and_O_and_G : MATLAB Function  TreatAsAtomicUnit=on
  THE_W_EFF_and_O_and_G : MATLAB Function  TreatAsAtomicUnit=on
  CALC_POS : Outport
  wires:
  Bus Selector/1 -> THE_W_EFF_and_O_and_G/4(theta1)  "<TH1>"
  Bus Selector/2 -> THE_W_EFF_and_O_and_G/5(theta2)  "<TH2>"
  Bus Selector/3 -> THE_W_EFF_and_O_and_G/6(theta3)  "<TH3>"
  Bus Selector/4 -> THE_W_EFF_and_O_and_G/7(theta4)  "<TH4>"
  Bus Creator/1 -> CALC_POS/1
  Constant18/1 -> THE_W_EFF_and_O_and_G/1(L1Y_s)
  Constant17/1 -> THE_W_EFF_and_O_and_G/2(L2Y_s)
  Constant19/1 -> THE_W_EFF_and_O_and_G/3(L3Y_s)
  THE_W_EFF_and_O_and_G/4(WF_pos_O3) -> Bus Creator/4  "WF_pos_O3"
  THE_W_EFF_and_O_and_G/6(WF_pos_G2) -> Bus Creator/6  "WF_pos_G2"
  THE_W_EFF_and_O_and_G/3(WF_pos_O2) -> Bus Creator/3  "WF_pos_O2"
  THE_W_EFF_and_O_and_G/7(WF_pos_G3) -> Bus Creator/7  "WF_pos_G3"
  THE_W_EFF_and_O_and_G/1(WF_pos_eff) -> Bus Creator/1  "WF_pos_EFF"
  THE_W_EFF_and_O_and_G/5(WF_pos_G1) -> Bus Creator/5  "WF_pos_G1"
  THE_W_EFF_and_O_and_G/2(WF_pos_O1) -> Bus Creator/2  "WF_pos_O1"
  MODEL_BUS/1 -> Bus Selector1/1, Bus Selector/1
  Bus Selector1/1 -> THE_A_EFF_and_O_and_G/4(theta1)  "<TH1>"
  Bus Selector1/2 -> THE_A_EFF_and_O_and_G/5(theta2)  "<TH2>"
  Bus Selector1/3 -> THE_A_EFF_and_O_and_G/6(theta3)  "<TH3>"
  Constant2/1 -> THE_A_EFF_and_O_and_G/1(L1Y_s)
  Constant1/1 -> THE_A_EFF_and_O_and_G/2(L2Y_s)
  Constant3/1 -> THE_A_EFF_and_O_and_G/3(L3Y_s)
  THE_A_EFF_and_O_and_G/7(AF_pos_G3) -> Bus Creator/14  "AF_pos_G3"
  THE_A_EFF_and_O_and_G/6(AF_pos_G2) -> Bus Creator/13  "AF_pos_G2"
  THE_A_EFF_and_O_and_G/5(AF_pos_G1) -> Bus Creator/12  "AF_pos_G1"
  THE_A_EFF_and_O_and_G/4(AF_pos_O3) -> Bus Creator/11  "AF_pos_O3"
  THE_A_EFF_and_O_and_G/3(AF_pos_O2) -> Bus Creator/10  "AF_pos_O2"
  THE_A_EFF_and_O_and_G/2(AF_pos_O1) -> Bus Creator/9  "AF_pos_O1"
  THE_A_EFF_and_O_and_G/1(AF_pos_eff) -> Bus Creator/8  "AF_pos_EFF"

== system bhzzz/Create_PLANT_BUS2/MEAS ==
  MODEL_BUS : Inport
  Bus Creator : BusCreator  Inputs=3
  Bus Selector : BusSelector  OutputSignals=TH1,TH2,TH3,TH4
  Bus Selector1 : BusSelector  OutputSignals=TH1_D,TH2_D,TH3_D,TH4_D
  Bus Selector2 : BusSelector  OutputSignals=TH1_DD,TH2_DD,TH3_DD,TH4_DD
  Mux : Mux
  Mux1 : Mux
  Mux2 : Mux
  Reshape : Reshape  OutputDimensionality=Column vector (2-D)
  Reshape1 : Reshape  OutputDimensionality=Column vector (2-D)
  Reshape2 : Reshape  OutputDimensionality=Column vector (2-D)
  MEAS : Outport
  wires:
  MODEL_BUS/1 -> Bus Selector/1, Bus Selector2/1, Bus Selector1/1
  Bus Selector/1 -> Mux/1  "<TH1>"
  Bus Selector/2 -> Mux/2  "<TH2>"
  Bus Selector/3 -> Mux/3  "<TH3>"
  Bus Selector/4 -> Mux/4  "<TH4>"
  Bus Selector1/1 -> Mux1/1  "<TH1_D>"
  Bus Selector1/2 -> Mux1/2  "<TH2_D>"
  Bus Selector1/3 -> Mux1/3  "<TH3_D>"
  Bus Selector1/4 -> Mux1/4  "<TH4_D>"
  Bus Selector2/1 -> Mux2/1  "<TH1_DD>"
  Bus Selector2/2 -> Mux2/2  "<TH2_DD>"
  Bus Selector2/3 -> Mux2/3  "<TH3_DD>"
  Bus Selector2/4 -> Mux2/4  "<TH4_DD>"
  Mux/1 -> Reshape/1  "TH_POS"
  Mux1/1 -> Reshape1/1  "TH_VEL"
  Mux2/1 -> Reshape2/1  "TH_ACC"
  Reshape/1 -> Bus Creator/1  "TH_POS"
  Reshape1/1 -> Bus Creator/2  "TH_VEL"
  Reshape2/1 -> Bus Creator/3  "TH_ACC"
  Bus Creator/1 -> MEAS/1

== system bhzzz/Create_PLANT_BUS2/Subsystem ==
  MODEL : Inport
  MEAS : Inport  Port=2
  CALC_POS : Inport  Port=3
  CALC_GRAV_TQ : Inport  Port=4
  Bus Creator : BusCreator  Inputs=4
  PLANT_B : Outport
  wires:
  MODEL/1 -> Bus Creator/1  "MODEL_BUS"
  MEAS/1 -> Bus Creator/2  "MEAS_BUS"
  CALC_POS/1 -> Bus Creator/3  "CALC_POS_BUS"
  Bus Creator/1 -> PLANT_B/1
  CALC_GRAV_TQ/1 -> Bus Creator/4  "CALC_GRAV_TQ_BUS"
